simulink model "METI_DTTH_PNT"  (R2018b)
settings: Solver=ode8  StartTime=0  StopTime=end_time  FixedStep=sampling_time  RelTol=1e-3
PreLoadFcn:
  | METI_DTTH_PNT_PreLoad;
undefined symbols (not defined in the file or in its folder): degC2K, DF_PNT_DFBlock2DFAir_Heat_Resi_KpW, DF_PNT_DFBlock_Heat_Capa_JpK, DF_PNT_DFBlock_Temp_ini_degC, DF_PNT_DFOil2DFBlock_Heat_Resi_KpW, DF_PNT_DFOil_Heat_Capa_JpK, DF_PNT_DFOil_Temp_ini_degC, DF_PNT_TMBlock2DFBlock_Heat_Resi_KpW, TM_PNT_CVTF2TMBlock_Heat_Resi_KpW, TM_PNT_CVTF_Heat_Capa_JpK, TM_PNT_CVTF_Temp_ini_degC, TM_PNT_ENGBlock2TMBlock_Heat_Resi_KpW, TM_PNT_TMBlock2TMAir_Heat_Resi_KpW, TM_PNT_TMBlock_Heat_Capa_JpK, TM_PNT_TMBlock_Temp_ini_degC
settings Model: Creator=nishimura  LastModifiedBy=E00026
settings DataIOCC: LimitDataPoints=on  SaveFormat=Array  SaveOutput=off  InspectSignalLogs=on  SaveTime=off
settings OptimizationCC: BlockReduction=off  BooleanDataType=off  LifeSpan=inf
settings DebuggingCC: SaveWithParameterizedLinksMsg=none  UnderspecifiedInitializationDetection=Classic  MergeDetectMultiDrivingBlocksExec=none  SignalResolutionControl=TryResolveAllWithWarning  StrictBusMsg=ErrorOnBusTreatedAsVector  SFUnexpectedBacktrackingDiag=warning  SFNoUnconditionalDefaultTransitionDiag=warning  SFExecutionAtInitializationDiag=none
settings HardwareCC: ProdBitPerPointer=32  ProdBitPerSizeT=32  ProdBitPerPtrDiffT=32  ProdLargestAtomicFloat=None  ProdIntDivRoundTo=Undefined  ProdEndianess=Unspecified  ProdWordSize=32  ProdHWDeviceType=32-bit Generic  TargetUnknown=on
settings ModelReferenceCC: PropagateSignalLabelsOutOfModel=off
settings SFSimCC: SimUseLocalCustomCode=off
settings RTWCC: RTWUseLocalCustomCode=off
settings CodeAppCC: StateflowObjectComments=on
settings GRTTargetCC: TargetLangStandard=C89/C90 (ANSI)  GeneratePreprocessorConditionals=Disable all
settings ConfigComp: CovMetricSettings=dw  CovHtmlReporting=on  CovSaveCumulativeToWorkspaceVar=on  CovSaveSingleToWorkspaceVar=on  CovExternalEMLEnable=off  CovSFcnEnable=off

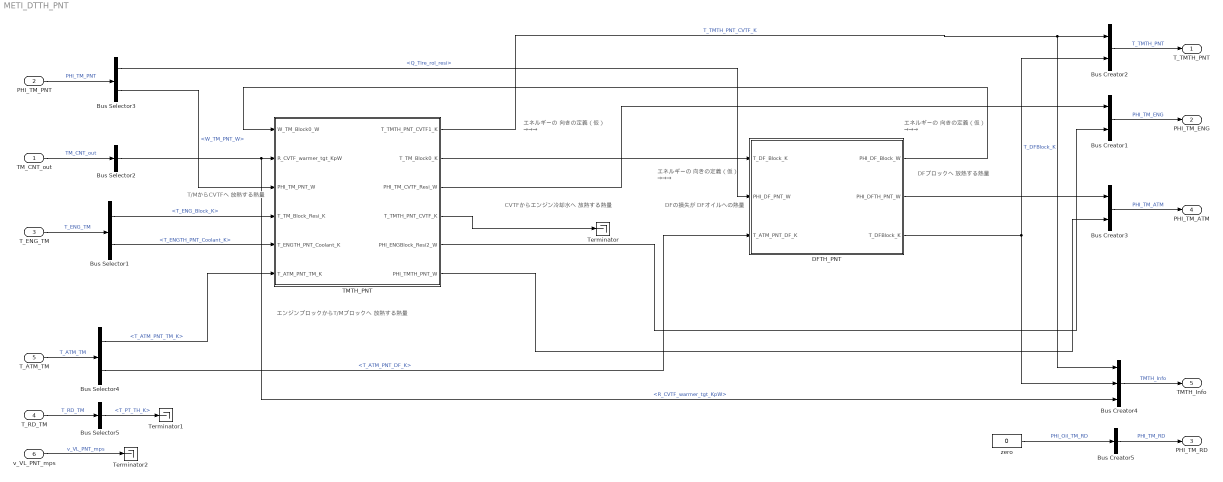
== system METI_DTTH_PNT ==
  note: DFブロックへ
      | 放熱する熱量
  note: CVTFからエンジン冷却水へ
      | 放熱する熱量
  note: エンジンブロックからT/Mブロックへ
      | 放熱する熱量
  note: エネルギーの
      | 向きの定義（仮）
      | →→→
  note: エネルギーの
      | 向きの定義（仮）
      | →→→
  note: エネルギーの
      | 向きの定義（仮）
      | →→→
  note: T/MからCVTFへ
      | 放熱する熱量
  note: DFの損失が
      | DFオイルへの熱量
  TM_CNT_out : Inport  OutDataTypeStr=Bus: slBus7_TM_CNT_out  SampleTime=[0.001,0]
      settings: AttributesFormatString=|
      | <SampleTime = %<SampleTime>>
      | <%<OutDataTypeStr>>
  PHI_TM_PNT : Inport  Port=2  OutDataTypeStr=Bus: slBus6_PHI_TM_PNT  SampleTime=0
      settings: AttributesFormatString=|
      | <SampleTime = %<SampleTime>>
      | <%<OutDataTypeStr>>
  T_ENG_TM : Inport  Port=3  OutDataTypeStr=Bus: slBus7_T_ENG_TM  SampleTime=0
      settings: AttributesFormatString=|
      | <SampleTime = %<SampleTime>>
      | <%<OutDataTypeStr>>
  T_RD_TM : Inport  Port=4  OutDataTypeStr=Bus: T_RD_TM
      settings: AttributesFormatString=|
      | <SampleTime = %<SampleTime>>
      | <%<OutDataTypeStr>>
  T_ATM_TM : Inport  Port=5  OutDataTypeStr=Bus: slBus8_T_ATM_TM
      settings: AttributesFormatString=|
      | <SampleTime = %<SampleTime>>
      | <%<OutDataTypeStr>>
  v_VL_PNT_mps : Inport  Port=6  OutDataTypeStr=double  PortDimensions=1  SampleTime=[0.001,0]
  Bus Creator1 : BusCreator  Inputs=2
  Bus Creator2 : BusCreator  Inputs=2
  Bus Creator3 : BusCreator  Inputs=2
  Bus Creator4 : BusCreator  Inputs=3
  Bus Creator5 : BusCreator  Inputs=1
  Bus Selector1 : BusSelector  OutputSignals=T_ENG_Block_K,T_ENGTH_PNT_Coolant_K
  Bus Selector2 : BusSelector  OutputSignals=R_CVTF_warmer_tgt_KpW
  Bus Selector3 : BusSelector  OutputSignals=Q_Tire_rol_resi,W_TM_PNT_W
  Bus Selector4 : BusSelector  OutputSignals=T_ATM_PNT_TM_K,T_ATM_PNT_DF_K
  Bus Selector5 : BusSelector  OutputSignals=T_PT_TH_K
  DFTH_PNT : Subsystem
      mask Display: image(imread('picture\回転変換.png'))
  TMTH_PNT : Subsystem
      mask Display: image(imread('picture\image\トランスミッション02.jpg'))
  Terminator : Terminator
  Terminator1 : Terminator
  Terminator2 : Terminator
  zero : Constant  Value=0
  T_TMTH_PNT : Outport  OutDataTypeStr=Bus: slBus9_T_TMTH_PNT  SampleTime=0
      settings: AttributesFormatString=<%<OutDataTypeStr>>
  PHI_TM_ENG : Outport  Port=2  OutDataTypeStr=Bus: slBus10_PHI_TM_ENG  SampleTime=0
      settings: AttributesFormatString=<%<OutDataTypeStr>>
  PHI_TM_RD : Outport  Port=3  OutDataTypeStr=Bus: slBus11_PHI_TM_RD
      settings: AttributesFormatString=<%<OutDataTypeStr>>
  PHI_TM_ATM : Outport  Port=4  OutDataTypeStr=Bus: slBus12_PHI_TM_ATM  SampleTime=0
      settings: AttributesFormatString=<%<OutDataTypeStr>>
  TMTH_Info : Outport  Port=5  OutDataTypeStr=Bus: slBus13_TMTH_Info
      settings: AttributesFormatString=<%<OutDataTypeStr>>
  wires:
  DFTH_PNT/2(PHI_DFTH_PNT_W) -> Bus Creator3/1
  Bus Selector4/2 -> DFTH_PNT/3(T_ATM_PNT_DF_K)  "<T_ATM_PNT_DF_K>"
  TMTH_PNT/4(T_TMTH_PNT_CVTF_K) -> Terminator/1
  TMTH_PNT/2(T_TM_Block0_K) -> DFTH_PNT/1(T_DF_Block_K)
  DFTH_PNT/1(PHI_DF_Block_W) -> TMTH_PNT/1(W_TM_Block0_W)
  TMTH_PNT/6(PHI_TMTH_PNT_W) -> Bus Creator3/2
  TMTH_PNT/5(PHI_ENGBlock_Resi2_W) -> Bus Creator1/2
  TMTH_PNT/3(PHI_TM_CVTF_Resi_W) -> Bus Creator1/1
  T_ENG_TM/1 -> Bus Selector1/1  "T_ENG_TM"
  Bus Selector1/1 -> TMTH_PNT/4(T_TM_Block_Resi_K)  "<T_ENG_Block_K>"
  Bus Selector1/2 -> TMTH_PNT/5(T_ENGTH_PNT_Coolant_K)  "<T_ENGTH_PNT_Coolant_K>"
  TMTH_PNT/1(T_TMTH_PNT_CVTF1_K) -> Bus Creator2/1, Bus Creator4/1  "T_TMTH_PNT_CVTF_K"
  DFTH_PNT/3(T_DFBlock_K) -> Bus Creator2/2, Bus Creator4/2  "T_DFBlock_K"
  Bus Creator2/1 -> T_TMTH_PNT/1  "T_TMTH_PNT"
  Bus Creator1/1 -> PHI_TM_ENG/1  "PHI_TM_ENG"
  Bus Creator3/1 -> PHI_TM_ATM/1  "PHI_TM_ATM"
  Bus Creator4/1 -> TMTH_Info/1  "TMTH_Info"
  PHI_TM_PNT/1 -> Bus Selector3/1  "PHI_TM_PNT"
  Bus Selector3/2 -> TMTH_PNT/3(PHI_TM_PNT_W)  "<W_TM_PNT_W>"
  Bus Selector3/1 -> DFTH_PNT/2(PHI_DF_PNT_W)  "<Q_Tire_rol_resi>"
  TM_CNT_out/1 -> Bus Selector2/1  "TM_CNT_out"
  Bus Selector2/1 -> TMTH_PNT/2(R_CVTF_warmer_tgt_KpW), Bus Creator4/3  "<R_CVTF_warmer_tgt_KpW>"
  T_ATM_TM/1 -> Bus Selector4/1  "T_ATM_TM"
  Bus Selector4/1 -> TMTH_PNT/6(T_ATM_PNT_TM_K)  "<T_ATM_PNT_TM_K>"
  Bus Creator5/1 -> PHI_TM_RD/1  "PHI_TM_RD"
  zero/1 -> Bus Creator5/1  "PHI_Oil_TM_RD"
  T_RD_TM/1 -> Bus Selector5/1  "T_RD_TM"
  Bus Selector5/1 -> Terminator1/1  "<T_PT_TH_K>"
  v_VL_PNT_mps/1 -> Terminator2/1  "v_VL_PNT_mps"

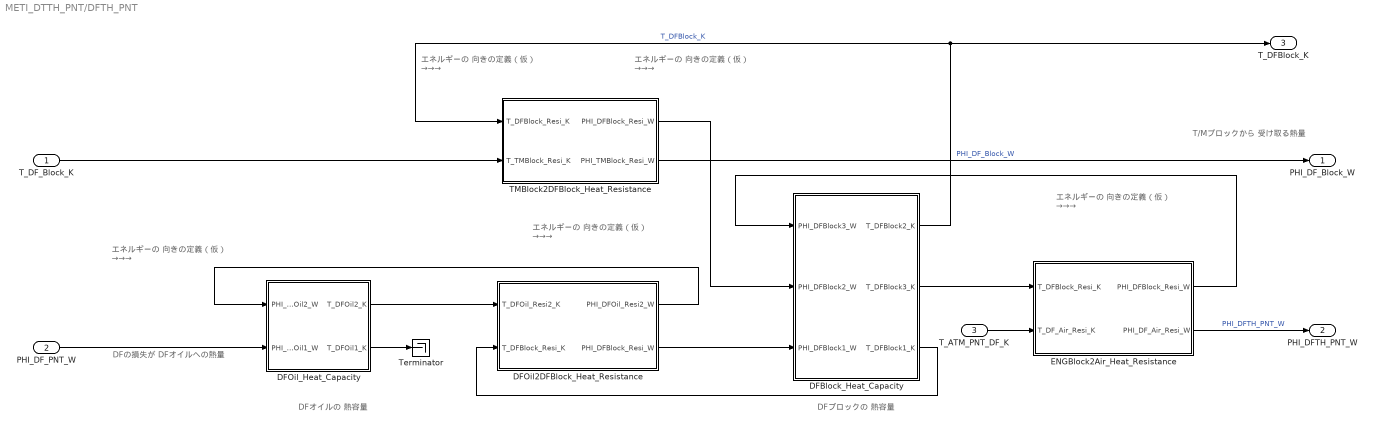
== system METI_DTTH_PNT/DFTH_PNT ==
  note: エネルギーの
      | 向きの定義（仮）
      | →→→
  note: エネルギーの
      | 向きの定義（仮）
      | →→→
  note: エネルギーの
      | 向きの定義（仮）
      | →→→
  note: エネルギーの
      | 向きの定義（仮）
      | →→→
  note: エネルギーの
      | 向きの定義（仮）
      | →→→
  note: DFの損失が
      | DFオイルへの熱量
  note: DFブロックの
      | 熱容量
  note: DFオイルの
      | 熱容量
  note: T/Mブロックから
      | 受け取る熱量
  T_DF_Block_K : Inport
  PHI_DF_PNT_W : Inport  Port=2
  T_ATM_PNT_DF_K : Inport  Port=3
  DFBlock_Heat_Capacity : Subsystem
  DFOil2DFBlock_Heat_Resistance : Subsystem
  DFOil_Heat_Capacity : Subsystem
  ENGBlock2Air_Heat_Resistance : Subsystem
  TMBlock2DFBlock_Heat_Resistance : Subsystem
  Terminator : Terminator
  PHI_DF_Block_W : Outport
  PHI_DFTH_PNT_W : Outport  Port=2
  T_DFBlock_K : Outport  Port=3
  wires:
  PHI_DF_PNT_W/1 -> DFOil_Heat_Capacity/2(PHI_DFOil1_W)
  DFOil_Heat_Capacity/2(T_DFOil1_K) -> Terminator/1
  DFBlock_Heat_Capacity/1(T_DFBlock2_K) -> TMBlock2DFBlock_Heat_Resistance/1(T_DFBlock_Resi_K), T_DFBlock_K/1  "T_DFBlock_K"
  TMBlock2DFBlock_Heat_Resistance/1(PHI_DFBlock_Resi_W) -> DFBlock_Heat_Capacity/2(PHI_DFBlock2_W)
  TMBlock2DFBlock_Heat_Resistance/2(PHI_TMBlock_Resi_W) -> PHI_DF_Block_W/1  "PHI_DF_Block_W"
  T_DF_Block_K/1 -> TMBlock2DFBlock_Heat_Resistance/2(T_TMBlock_Resi_K)
  ENGBlock2Air_Heat_Resistance/2(PHI_DF_Air_Resi_W) -> PHI_DFTH_PNT_W/1  "PHI_DFTH_PNT_W"
  T_ATM_PNT_DF_K/1 -> ENGBlock2Air_Heat_Resistance/2(T_DF_Air_Resi_K)
  DFBlock_Heat_Capacity/2(T_DFBlock3_K) -> ENGBlock2Air_Heat_Resistance/1(T_DFBlock_Resi_K)
  ENGBlock2Air_Heat_Resistance/1(PHI_DFBlock_Resi_W) -> DFBlock_Heat_Capacity/1(PHI_DFBlock3_W)
  DFOil2DFBlock_Heat_Resistance/2(PHI_DFBlock_Resi_W) -> DFBlock_Heat_Capacity/3(PHI_DFBlock1_W)
  DFBlock_Heat_Capacity/3(T_DFBlock1_K) -> DFOil2DFBlock_Heat_Resistance/2(T_DFBlock_Resi_K)
  DFOil2DFBlock_Heat_Resistance/1(PHI_DFOil_Resi2_W) -> DFOil_Heat_Capacity/1(PHI_DFOil2_W)
  DFOil_Heat_Capacity/1(T_DFOil2_K) -> DFOil2DFBlock_Heat_Resistance/1(T_DFOil_Resi2_K)

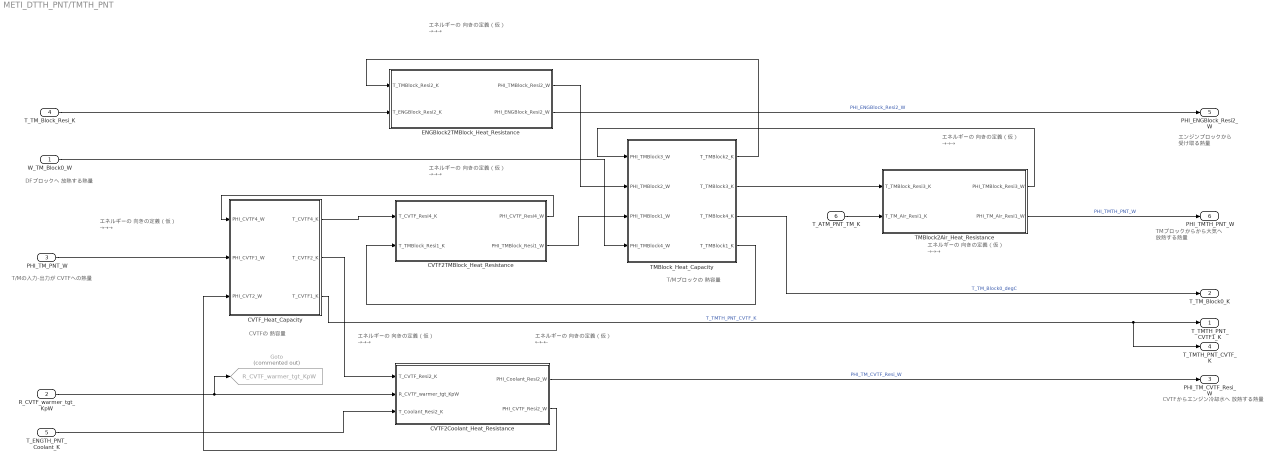
== system METI_DTTH_PNT/TMTH_PNT ==
  note: TMブロックからから大気へ
      | 放熱する熱量
  note: エネルギーの
      | 向きの定義（仮）
      | →→→
  note: エネルギーの
      | 向きの定義（仮）
      | →→→
  note: エネルギーの
      | 向きの定義（仮）
      | →→→
  note: エネルギーの
      | 向きの定義（仮）
      | →→→
  note: エネルギーの
      | 向きの定義（仮）
      | →→→
  note: エネルギーの
      | 向きの定義（仮）
      | →→→
  note: エネルギーの
      | 向きの定義（仮）
      | ←←←
  note: T/Mの入力-出力が
      | CVTFへの熱量
  note: CVTFからエンジン冷却水へ
      | 放熱する熱量
  note: エンジンブロックから
      | 受け取る熱量
  note: DFブロックへ
      | 放熱する熱量
  note: T/Mブロックの
      | 熱容量
  note: CVTFの
      | 熱容量
  W_TM_Block0_W : Inport
  R_CVTF_warmer_tgt_KpW : Inport  Port=2
  PHI_TM_PNT_W : Inport  Port=3
  T_TM_Block_Resi_K : Inport  Port=4
  T_ENGTH_PNT_Coolant_K : Inport  Port=5
  T_ATM_PNT_TM_K : Inport  Port=6
  CVTF2Coolant_Heat_Resistance : Subsystem
  CVTF2TMBlock_Heat_Resistance : Subsystem
  CVTF_Heat_Capacity : Subsystem
  ENGBlock2TMBlock_Heat_Resistance : Subsystem
  Goto : Goto  Commented=on  GotoTag=R_CVTF_warmer_tgt_KpW  TagVisibility=global
  TMBlock2Air_Heat_Resistance : Subsystem
  TMBlock_Heat_Capacity : Subsystem
  T_TMTH_PNT_CVTF1_K : Outport
  T_TM_Block0_K : Outport  Port=2
  PHI_TM_CVTF_Resi_W : Outport  Port=3
  T_TMTH_PNT_CVTF_K : Outport  Port=4
  PHI_ENGBlock_Resi2_W : Outport  Port=5
  PHI_TMTH_PNT_W : Outport  Port=6
  wires:
  R_CVTF_warmer_tgt_KpW/1 -> Goto/1, CVTF2Coolant_Heat_Resistance/2(R_CVTF_warmer_tgt_KpW)
  W_TM_Block0_W/1 -> TMBlock_Heat_Capacity/4(PHI_TMBlock4_W)
  TMBlock_Heat_Capacity/3(T_TMBlock4_K) -> T_TM_Block0_K/1  "T_TM_Block0_degC"
  TMBlock_Heat_Capacity/1(T_TMBlock2_K) -> ENGBlock2TMBlock_Heat_Resistance/1(T_TMBlock_Resi2_K)
  ENGBlock2TMBlock_Heat_Resistance/1(PHI_TMBlock_Resi2_W) -> TMBlock_Heat_Capacity/2(PHI_TMBlock2_W)
  T_ENGTH_PNT_Coolant_K/1 -> CVTF2Coolant_Heat_Resistance/3(T_Coolant_Resi2_K)
  CVTF2Coolant_Heat_Resistance/1(PHI_Coolant_Resi2_W) -> PHI_TM_CVTF_Resi_W/1  "PHI_TM_CVTF_Resi_W"
  CVTF2Coolant_Heat_Resistance/2(PHI_CVTF_Resi2_W) -> CVTF_Heat_Capacity/3(PHI_CVT2_W)
  CVTF_Heat_Capacity/2(T_CVTF2_K) -> CVTF2Coolant_Heat_Resistance/1(T_CVTF_Resi2_K)
  ENGBlock2TMBlock_Heat_Resistance/2(PHI_ENGBlock_Resi2_W) -> PHI_ENGBlock_Resi2_W/1  "PHI_ENGBlock_Resi2_W"
  T_TM_Block_Resi_K/1 -> ENGBlock2TMBlock_Heat_Resistance/2(T_ENGBlock_Resi2_K)
  TMBlock2Air_Heat_Resistance/2(PHI_TM_Air_Resi1_W) -> PHI_TMTH_PNT_W/1  "PHI_TMTH_PNT_W"
  T_ATM_PNT_TM_K/1 -> TMBlock2Air_Heat_Resistance/2(T_TM_Air_Resi1_K)
  TMBlock_Heat_Capacity/2(T_TMBlock3_K) -> TMBlock2Air_Heat_Resistance/1(T_TMBlock_Resi3_K)
  TMBlock2Air_Heat_Resistance/1(PHI_TMBlock_Resi3_W) -> TMBlock_Heat_Capacity/1(PHI_TMBlock3_W)
  PHI_TM_PNT_W/1 -> CVTF_Heat_Capacity/2(PHI_CVTF1_W)
  CVTF_Heat_Capacity/3(T_CVTF1_K) -> T_TMTH_PNT_CVTF1_K/1, T_TMTH_PNT_CVTF_K/1  "T_TMTH_PNT_CVTF_K"
  CVTF2TMBlock_Heat_Resistance/2(PHI_TMBlock_Resi1_W) -> TMBlock_Heat_Capacity/3(PHI_TMBlock1_W)
  TMBlock_Heat_Capacity/4(T_TMBlock1_K) -> CVTF2TMBlock_Heat_Resistance/2(T_TMBlock_Resi1_K)
  CVTF2TMBlock_Heat_Resistance/1(PHI_CVTF_Resi4_W) -> CVTF_Heat_Capacity/1(PHI_CVTF4_W)
  CVTF_Heat_Capacity/1(T_CVTF4_K) -> CVTF2TMBlock_Heat_Resistance/1(T_CVTF_Resi4_K)

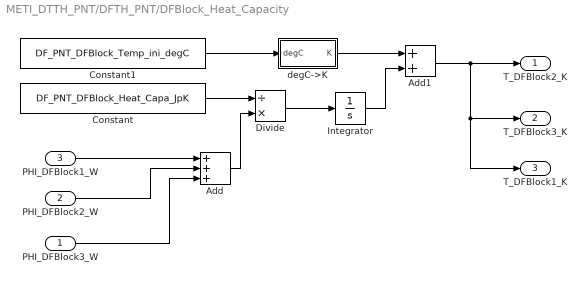
== system METI_DTTH_PNT/DFTH_PNT/DFBlock_Heat_Capacity ==
  PHI_DFBlock3_W : Inport
  PHI_DFBlock2_W : Inport  Port=2
  PHI_DFBlock1_W : Inport  Port=3
  Add : Sum  Inputs=+++
  Add1 : Sum
  Constant : Constant  Value=DF_PNT_DFBlock_Heat_Capa_JpK
  Constant1 : Constant  Value=DF_PNT_DFBlock_Temp_ini_degC
  Divide : Product  Inputs=/*
  Integrator : Integrator
  degC->K : Subsystem
  T_DFBlock2_K : Outport
  T_DFBlock3_K : Outport  Port=2
  T_DFBlock1_K : Outport  Port=3
  wires:
  degC->K/1(K) -> Add1/1
  Constant1/1 -> degC->K/1(degC)
  PHI_DFBlock3_W/1 -> Add/3
  PHI_DFBlock2_W/1 -> Add/2
  Add1/1 -> T_DFBlock2_K/1, T_DFBlock3_K/1, T_DFBlock1_K/1
  Integrator/1 -> Add1/2
  Divide/1 -> Integrator/1
  Add/1 -> Divide/2
  Constant/1 -> Divide/1
  PHI_DFBlock1_W/1 -> Add/1

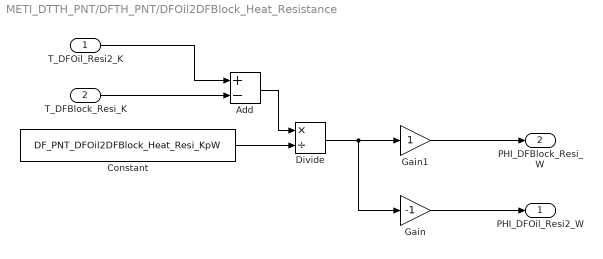
== system METI_DTTH_PNT/DFTH_PNT/DFOil2DFBlock_Heat_Resistance ==
  T_DFOil_Resi2_K : Inport
  T_DFBlock_Resi_K : Inport  Port=2
  Add : Sum  Inputs=+-
  Constant : Constant  Value=DF_PNT_DFOil2DFBlock_Heat_Resi_KpW
  Divide : Product  Inputs=*/
  Gain : Gain  Gain=-1
  Gain1 : Gain
  PHI_DFOil_Resi2_W : Outport
  PHI_DFBlock_Resi_W : Outport  Port=2
  wires:
  Gain1/1 -> PHI_DFBlock_Resi_W/1
  T_DFBlock_Resi_K/1 -> Add/2
  T_DFOil_Resi2_K/1 -> Add/1
  Gain/1 -> PHI_DFOil_Resi2_W/1
  Divide/1 -> Gain1/1, Gain/1
  Add/1 -> Divide/1
  Constant/1 -> Divide/2

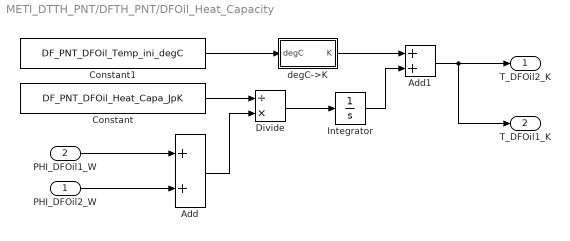
== system METI_DTTH_PNT/DFTH_PNT/DFOil_Heat_Capacity ==
  PHI_DFOil2_W : Inport
  PHI_DFOil1_W : Inport  Port=2
  Add : Sum
  Add1 : Sum
  Constant : Constant  Value=DF_PNT_DFOil_Heat_Capa_JpK
  Constant1 : Constant  Value=DF_PNT_DFOil_Temp_ini_degC
  Divide : Product  Inputs=/*
  Integrator : Integrator
  degC->K : Subsystem
  T_DFOil2_K : Outport
  T_DFOil1_K : Outport  Port=2
  wires:
  degC->K/1(K) -> Add1/1
  Constant1/1 -> degC->K/1(degC)
  Add1/1 -> T_DFOil2_K/1, T_DFOil1_K/1
  Integrator/1 -> Add1/2
  Divide/1 -> Integrator/1
  Add/1 -> Divide/2
  Constant/1 -> Divide/1
  PHI_DFOil1_W/1 -> Add/1
  PHI_DFOil2_W/1 -> Add/2

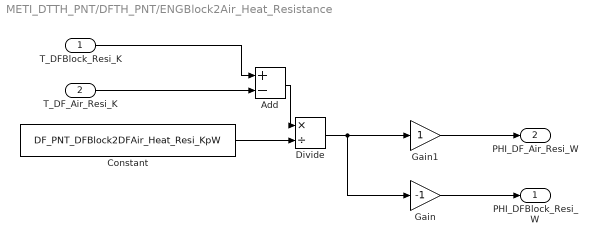
== system METI_DTTH_PNT/DFTH_PNT/ENGBlock2Air_Heat_Resistance ==
  T_DFBlock_Resi_K : Inport
  T_DF_Air_Resi_K : Inport  Port=2
  Add : Sum  Inputs=+-
  Constant : Constant  Value=DF_PNT_DFBlock2DFAir_Heat_Resi_KpW
  Divide : Product  Inputs=*/
  Gain : Gain  Gain=-1
  Gain1 : Gain
  PHI_DFBlock_Resi_W : Outport
  PHI_DF_Air_Resi_W : Outport  Port=2
  wires:
  Gain1/1 -> PHI_DF_Air_Resi_W/1
  T_DF_Air_Resi_K/1 -> Add/2
  T_DFBlock_Resi_K/1 -> Add/1
  Gain/1 -> PHI_DFBlock_Resi_W/1
  Divide/1 -> Gain1/1, Gain/1
  Add/1 -> Divide/1
  Constant/1 -> Divide/2

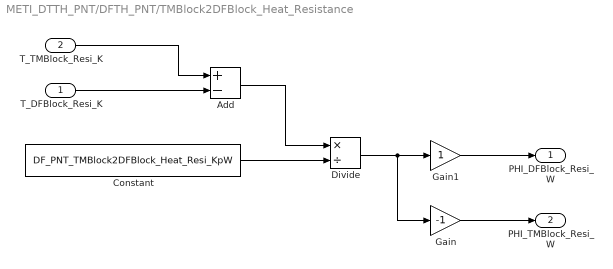
== system METI_DTTH_PNT/DFTH_PNT/TMBlock2DFBlock_Heat_Resistance ==
  T_DFBlock_Resi_K : Inport
  T_TMBlock_Resi_K : Inport  Port=2
  Add : Sum  Inputs=+-
  Constant : Constant  Value=DF_PNT_TMBlock2DFBlock_Heat_Resi_KpW
  Divide : Product  Inputs=*/
  Gain : Gain  Gain=-1
  Gain1 : Gain
  PHI_DFBlock_Resi_W : Outport
  PHI_TMBlock_Resi_W : Outport  Port=2
  wires:
  Gain1/1 -> PHI_DFBlock_Resi_W/1
  T_DFBlock_Resi_K/1 -> Add/2
  T_TMBlock_Resi_K/1 -> Add/1
  Gain/1 -> PHI_TMBlock_Resi_W/1
  Divide/1 -> Gain1/1, Gain/1
  Add/1 -> Divide/1
  Constant/1 -> Divide/2

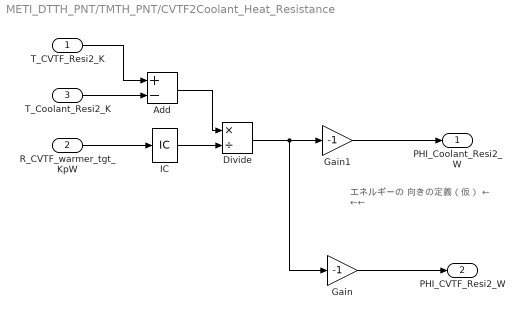
== system METI_DTTH_PNT/TMTH_PNT/CVTF2Coolant_Heat_Resistance ==
  note: エネルギーの
      | 向きの定義（仮）
      | ← ←←
  T_CVTF_Resi2_K : Inport
  R_CVTF_warmer_tgt_KpW : Inport  Port=2
  T_Coolant_Resi2_K : Inport  Port=3
  Add : Sum  Inputs=+-
  Divide : Product  Inputs=*/
  Gain : Gain  Gain=-1
  Gain1 : Gain  Gain=-1
  IC : InitialCondition  Value=0.1
  PHI_Coolant_Resi2_W : Outport
  PHI_CVTF_Resi2_W : Outport  Port=2
  wires:
  R_CVTF_warmer_tgt_KpW/1 -> IC/1
  IC/1 -> Divide/2
  Gain1/1 -> PHI_Coolant_Resi2_W/1
  Gain/1 -> PHI_CVTF_Resi2_W/1
  T_CVTF_Resi2_K/1 -> Add/1
  T_Coolant_Resi2_K/1 -> Add/2
  Divide/1 -> Gain1/1, Gain/1
  Add/1 -> Divide/1

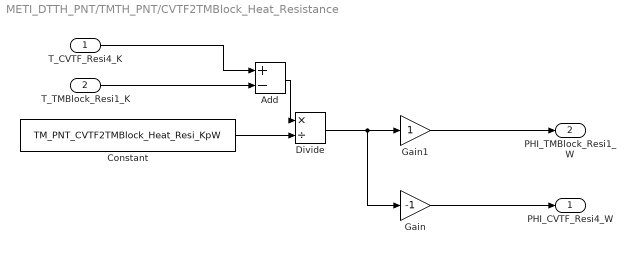
== system METI_DTTH_PNT/TMTH_PNT/CVTF2TMBlock_Heat_Resistance ==
  T_CVTF_Resi4_K : Inport
  T_TMBlock_Resi1_K : Inport  Port=2
  Add : Sum  Inputs=+-
  Constant : Constant  Value=TM_PNT_CVTF2TMBlock_Heat_Resi_KpW
  Divide : Product  Inputs=*/
  Gain : Gain  Gain=-1
  Gain1 : Gain
  PHI_CVTF_Resi4_W : Outport
  PHI_TMBlock_Resi1_W : Outport  Port=2
  wires:
  Gain1/1 -> PHI_TMBlock_Resi1_W/1
  T_TMBlock_Resi1_K/1 -> Add/2
  T_CVTF_Resi4_K/1 -> Add/1
  Gain/1 -> PHI_CVTF_Resi4_W/1
  Divide/1 -> Gain1/1, Gain/1
  Add/1 -> Divide/1
  Constant/1 -> Divide/2

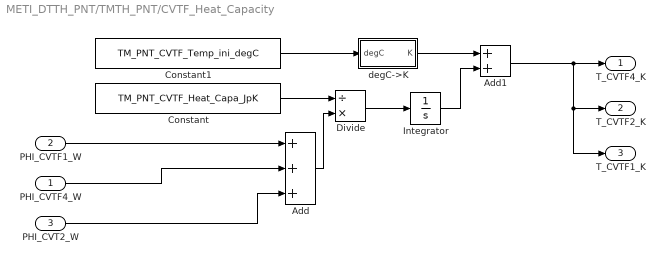
== system METI_DTTH_PNT/TMTH_PNT/CVTF_Heat_Capacity ==
  PHI_CVTF4_W : Inport
  PHI_CVTF1_W : Inport  Port=2
  PHI_CVT2_W : Inport  Port=3
  Add : Sum  Inputs=+++
  Add1 : Sum
  Constant : Constant  Value=TM_PNT_CVTF_Heat_Capa_JpK
  Constant1 : Constant  Value=TM_PNT_CVTF_Temp_ini_degC
  Divide : Product  Inputs=/*
  Integrator : Integrator
  degC->K : Subsystem
  T_CVTF4_K : Outport
  T_CVTF2_K : Outport  Port=2
  T_CVTF1_K : Outport  Port=3
  wires:
  degC->K/1(K) -> Add1/1
  Constant1/1 -> degC->K/1(degC)
  PHI_CVTF4_W/1 -> Add/2
  Add1/1 -> T_CVTF4_K/1, T_CVTF2_K/1, T_CVTF1_K/1
  Integrator/1 -> Add1/2
  Divide/1 -> Integrator/1
  Add/1 -> Divide/2
  Constant/1 -> Divide/1
  PHI_CVTF1_W/1 -> Add/1
  PHI_CVT2_W/1 -> Add/3

== system METI_DTTH_PNT/TMTH_PNT/ENGBlock2TMBlock_Heat_Resistance ==
  T_TMBlock_Resi2_K : Inport
  T_ENGBlock_Resi2_K : Inport  Port=2
  Add : Sum  Inputs=+-
  Constant : Constant  Value=TM_PNT_ENGBlock2TMBlock_Heat_Resi_KpW
  Divide : Product  Inputs=*/
  Gain : Gain  Gain=-1
  Gain1 : Gain
  PHI_TMBlock_Resi2_W : Outport
  PHI_ENGBlock_Resi2_W : Outport  Port=2
  wires:
  Gain1/1 -> PHI_TMBlock_Resi2_W/1
  T_TMBlock_Resi2_K/1 -> Add/2
  T_ENGBlock_Resi2_K/1 -> Add/1
  Gain/1 -> PHI_ENGBlock_Resi2_W/1
  Divide/1 -> Gain/1, Gain1/1
  Add/1 -> Divide/1
  Constant/1 -> Divide/2

== system METI_DTTH_PNT/TMTH_PNT/TMBlock2Air_Heat_Resistance ==
  T_TMBlock_Resi3_K : Inport
  T_TM_Air_Resi1_K : Inport  Port=2
  Add : Sum  Inputs=+-
  Constant : Constant  Value=TM_PNT_TMBlock2TMAir_Heat_Resi_KpW
  Divide : Product  Inputs=*/
  Gain : Gain  Gain=-1
  Gain1 : Gain
  PHI_TMBlock_Resi3_W : Outport
  PHI_TM_Air_Resi1_W : Outport  Port=2
  wires:
  Gain1/1 -> PHI_TM_Air_Resi1_W/1
  T_TM_Air_Resi1_K/1 -> Add/2
  T_TMBlock_Resi3_K/1 -> Add/1
  Gain/1 -> PHI_TMBlock_Resi3_W/1
  Divide/1 -> Gain1/1, Gain/1
  Add/1 -> Divide/1
  Constant/1 -> Divide/2

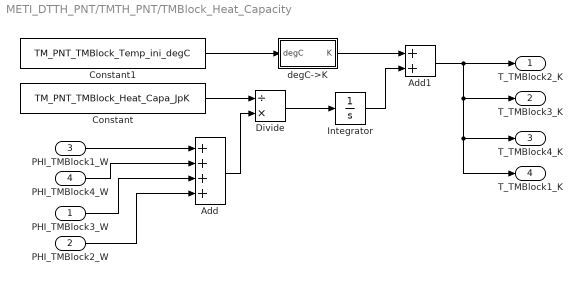
== system METI_DTTH_PNT/TMTH_PNT/TMBlock_Heat_Capacity ==
  PHI_TMBlock3_W : Inport
  PHI_TMBlock2_W : Inport  Port=2
  PHI_TMBlock1_W : Inport  Port=3
  PHI_TMBlock4_W : Inport  Port=4
  Add : Sum  Inputs=++++
  Add1 : Sum
  Constant : Constant  Value=TM_PNT_TMBlock_Heat_Capa_JpK
  Constant1 : Constant  Value=TM_PNT_TMBlock_Temp_ini_degC
  Divide : Product  Inputs=/*
  Integrator : Integrator
  degC->K : Subsystem
  T_TMBlock2_K : Outport
  T_TMBlock3_K : Outport  Port=2
  T_TMBlock4_K : Outport  Port=3
  T_TMBlock1_K : Outport  Port=4
  wires:
  degC->K/1(K) -> Add1/1
  Constant1/1 -> degC->K/1(degC)
  Add1/1 -> T_TMBlock2_K/1, T_TMBlock3_K/1, T_TMBlock4_K/1, T_TMBlock1_K/1
  PHI_TMBlock4_W/1 -> Add/2
  PHI_TMBlock3_W/1 -> Add/3
  Integrator/1 -> Add1/2
  Divide/1 -> Integrator/1
  Add/1 -> Divide/2
  Constant/1 -> Divide/1
  PHI_TMBlock1_W/1 -> Add/1
  PHI_TMBlock2_W/1 -> Add/4

== system METI_DTTH_PNT/DFTH_PNT/DFBlock_Heat_Capacity/degC->K ==
  degC : Inport
  Constant2 : Constant  Value=degC2K
  Sum : Sum  Inputs=++|
  K : Outport
  wires:
  Sum/1 -> K/1
  Constant2/1 -> Sum/1
  degC/1 -> Sum/2

== system METI_DTTH_PNT/DFTH_PNT/DFOil_Heat_Capacity/degC->K ==
  degC : Inport
  Constant2 : Constant  Value=degC2K
  Sum : Sum  Inputs=++|
  K : Outport
  wires:
  Sum/1 -> K/1
  Constant2/1 -> Sum/1
  degC/1 -> Sum/2

== system METI_DTTH_PNT/TMTH_PNT/CVTF_Heat_Capacity/degC->K ==
  degC : Inport
  Constant2 : Constant  Value=degC2K
  Sum : Sum  Inputs=++|
  K : Outport
  wires:
  Sum/1 -> K/1
  Constant2/1 -> Sum/1
  degC/1 -> Sum/2

== system METI_DTTH_PNT/TMTH_PNT/TMBlock_Heat_Capacity/degC->K ==
  degC : Inport
  Constant2 : Constant  Value=degC2K
  Sum : Sum  Inputs=++|
  K : Outport
  wires:
  Sum/1 -> K/1
  Constant2/1 -> Sum/1
  degC/1 -> Sum/2
